simulink model "Detection_subsystem"  (R2016a)
settings: Solver=VariableStepAuto  StartTime=0.0  StopTime=10.0  RelTol=1e-3
libraries: audiosources x6
settings Model: Creator=hi  LastModifiedBy=hi

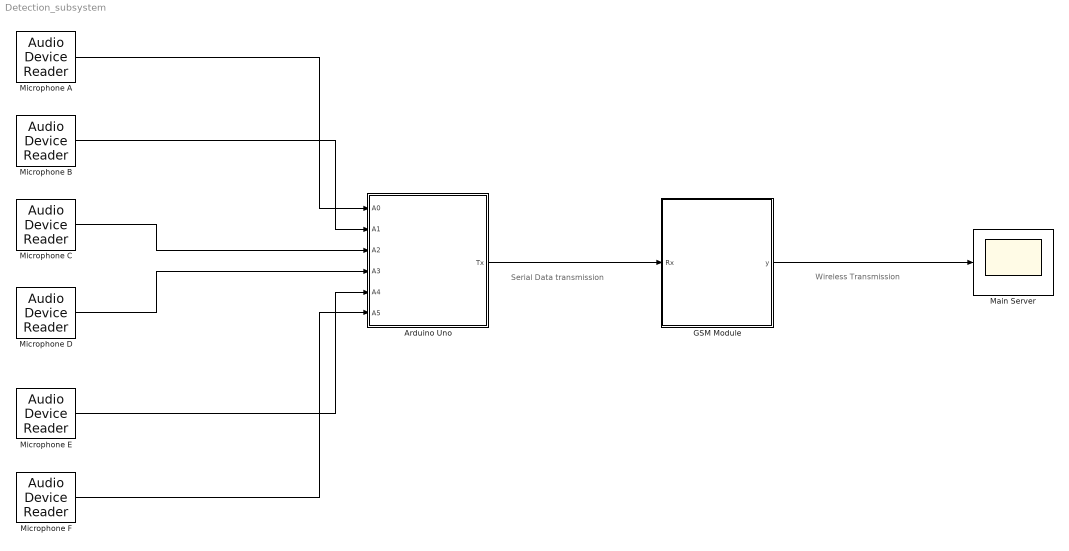
== system Detection_subsystem ==
  note: Wireless Transmission
  note: Serial Data transmission
  Arduino Uno : MATLAB Function  TreatAsAtomicUnit=on
  GSM Module : MATLAB Function  TreatAsAtomicUnit=on
  Main Server : Scope
  "Microphone A " : audiosources/Audio Device Reader  Driver=DirectSound  Device=Default  SampleRate=44100  NumChannels=1  SamplesPerFrame=1024  BitDepth=16-bit integer  NumBuffers=10  DefaultInputChannelMapping=on  InputChannelMapping=1:2  OutputNumOverrunSamples=off  OutputDataType=double  DriverIdx=1  DeviceWarnFlag=''
  Microphone B : audiosources/Audio Device Reader  Driver=DirectSound  Device=Default  SampleRate=44100  NumChannels=1  SamplesPerFrame=1024  BitDepth=16-bit integer  NumBuffers=10  DefaultInputChannelMapping=on  InputChannelMapping=1:2  OutputNumOverrunSamples=off  OutputDataType=double  DriverIdx=1  DeviceWarnFlag=''
  Microphone C : audiosources/Audio Device Reader  Driver=DirectSound  Device=Default  SampleRate=44100  NumChannels=1  SamplesPerFrame=1024  BitDepth=16-bit integer  NumBuffers=10  DefaultInputChannelMapping=on  InputChannelMapping=1:2  OutputNumOverrunSamples=off  OutputDataType=double  DriverIdx=1  DeviceWarnFlag=''
  Microphone D : audiosources/Audio Device Reader  Driver=DirectSound  Device=Default  SampleRate=44100  NumChannels=1  SamplesPerFrame=1024  BitDepth=16-bit integer  NumBuffers=10  DefaultInputChannelMapping=on  InputChannelMapping=1:2  OutputNumOverrunSamples=off  OutputDataType=double  DriverIdx=1  DeviceWarnFlag=''
  Microphone E : audiosources/Audio Device Reader  Driver=DirectSound  Device=Default  SampleRate=44100  NumChannels=1  SamplesPerFrame=1024  BitDepth=16-bit integer  NumBuffers=10  DefaultInputChannelMapping=on  InputChannelMapping=1:2  OutputNumOverrunSamples=off  OutputDataType=double  DriverIdx=1  DeviceWarnFlag=''
  Microphone F : audiosources/Audio Device Reader  Driver=DirectSound  Device=Default  SampleRate=44100  NumChannels=1  SamplesPerFrame=1024  BitDepth=16-bit integer  NumBuffers=10  DefaultInputChannelMapping=on  InputChannelMapping=1:2  OutputNumOverrunSamples=off  OutputDataType=double  DriverIdx=1  DeviceWarnFlag=''
  wires:
  "Microphone A "/1 -> Arduino Uno/1(A0)
  Microphone B/1 -> Arduino Uno/2(A1)
  Microphone C/1 -> Arduino Uno/3(A2)
  Microphone D/1 -> Arduino Uno/4(A3)
  Microphone F/1 -> Arduino Uno/6(A5)
  Microphone E/1 -> Arduino Uno/5(A4)
  GSM Module/1(y) -> Main Server/1
  Arduino Uno/1(Tx) -> GSM Module/1(Rx)

== matlab function Detection_subsystem/Arduino Uno ==
  data: A0 input; Tx output; A1 input; A2 input; A3 input; A4 input; A5 input
function Tx  = fcn(A0,A1,A2,A3,A4,A5)
%#codegen
  while(i<=1000)
  {min_1 = min(A0,min_1);
   max_1 = max(A0,max_1);
   min_2 = min(A1,min_2);
   max_2 = max(A1,max_2);
   min_3 = min(A2,min_3);
   max_3 = max(A2,max_3);
   min_4 = min(A3,min_4);
   max_4 = max(A3,max_4);
   min_5 = min(A4,min_5);
   max_5 = max(A4,max_5);
   min_6 = min(A5,min_6);
   max_6 = max(A5,max_6);
   i++;
   }
       i=0; 
       a[0] = max_1-min1;
       a[1] = max_2-min2;
       a[2] = max_3-min3;
       a[3] = max_4-min4;
       a[4] = max_5-min5;
       a[5]= max_6-min6;
       
       for(j=0;j=<5;j++)
           y=a[i];

== matlab function Detection_subsystem/GSM Module ==
  data: Rx input; y output
function y = fcn(Rx)
%#codegen

y = u;
